simulink model "NonSimplifiedMBFRC"  (R2023b)
settings: Solver=FixedStepAuto  StartTime=0.0  StopTime=t(end)  FixedStep=0.001  MaxStep=0.001  RelTol=1e-3
values from neighbouring files (symbols this model uses):
  a = 0.02+(j-1)*0.02    [MBFRC_ForLoops.m]    (also in Main.m = 0.001)
  f = f3    [MBFRC_ForLoops.m]    (also in Main.m = [0 freqs(1:Nfreqs)])
  phi_mat = zeros(2*length(f))    [MBFRC_ForLoops.m]    (also in Main.m)
  pQ = nQ    (= 12)    [MBFRC_ForLoops.m]    (also in Main.m)
  refOn = 1    [MBFRC_ForLoops.m]    (also in Main.m)
  tradRC_on = 1    [Main.m]
undefined symbols (not defined in the file or in its folder): phd, r_scale, tau
libraries: cstblocks x5
settings Model: Creator=maxja  LastModifiedBy=maxja

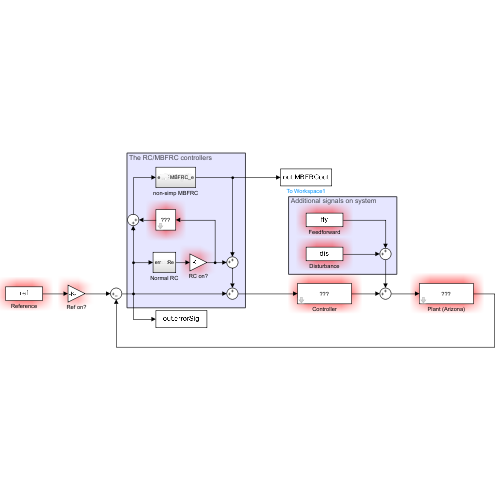
[thumbnail: Simulink's stored preview of the top-level diagram]
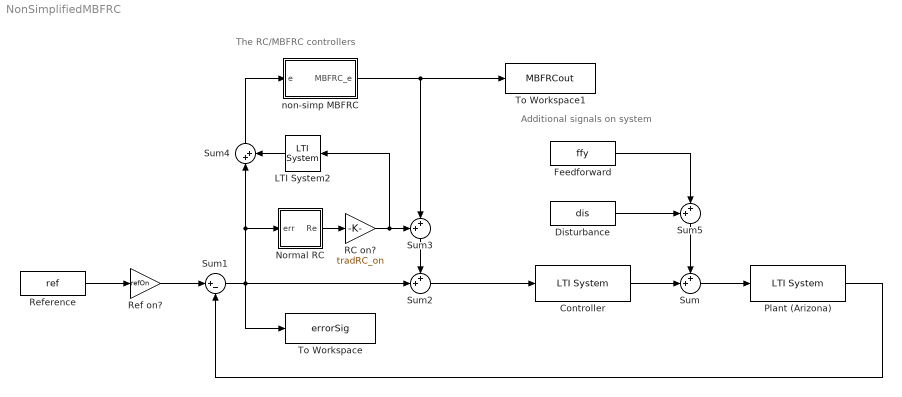
== system NonSimplifiedMBFRC ==
  note: Additional signals on system
  note: The RC/MBFRC controllers
  Controller : cstblocks/LTI System  sys=Cz  IC=[]  PadeOrder=0
  Disturbance : FromWorkspace  VariableName=dis
  Feedforward : FromWorkspace  VariableName=ffy
  LTI System2 : cstblocks/LTI System  sys=T  IC=[]  PadeOrder=0
  Normal RC : Subsystem
  Plant (Arizona) : cstblocks/LTI System  sys=Pz  IC=[]  PadeOrder=0
  RC on? : Gain  Gain=tradRC_on
  Ref on? : Gain  Gain=refOn
  Reference : FromWorkspace  VariableName=ref
  Sum{,2..3,5} (4 alike) : Sum  Inputs=++|
  Sum1 : Sum  Inputs=|+-
  Sum4 : Sum  Inputs=|++
  To Workspace : ToWorkspace  VariableName=errorSig  SaveFormat=Timeseries  SampleTime=-1
  To Workspace1 : ToWorkspace  VariableName=MBFRCout  SaveFormat=Timeseries  SampleTime=-1
  non-simp MBFRC : Subsystem
  wires:
  Controller/1 -> Sum/2
  Reference/1 -> Ref on?/1
  Plant (Arizona)/1 -> Sum1/2
  Sum2/1 -> Controller/1
  non-simp MBFRC/1(MBFRC_e) -> Sum3/2, To Workspace1/1
  LTI System2/1 -> Sum4/2
  Sum4/1 -> non-simp MBFRC/1(e)
  Normal RC/1(Re) -> RC on?/1
  Sum1/1 -> To Workspace/1, Sum2/2, Sum4/1, Normal RC/1(err)
  Sum3/1 -> Sum2/1
  Sum/1 -> Plant (Arizona)/1
  Disturbance/1 -> Sum5/1
  Ref on?/1 -> Sum1/1
  Feedforward/1 -> Sum5/2
  Sum5/1 -> Sum/1
  RC on?/1 -> Sum3/1, LTI System2/1

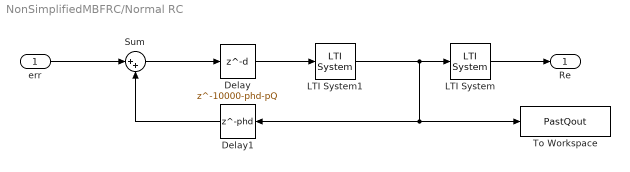
== system NonSimplifiedMBFRC/Normal RC ==
  err : Inport
  Delay : Delay  DelayLength=10000-phd-pQ
  Delay1 : Delay  DelayLength=phd
  LTI System : cstblocks/LTI System  sys=Lc  IC=[]  PadeOrder=0
  LTI System1 : cstblocks/LTI System  sys=Qc  IC=[]  PadeOrder=0
  Sum : Sum  Inputs=|++
  To Workspace : ToWorkspace  VariableName=PastQout  SaveFormat=Timeseries  SampleTime=-1
  Re : Outport
  wires:
  err/1 -> Sum/1
  Sum/1 -> Delay/1
  Delay/1 -> LTI System1/1
  LTI System/1 -> Re/1
  Delay1/1 -> Sum/2
  LTI System1/1 -> To Workspace/1, Delay1/1, LTI System/1

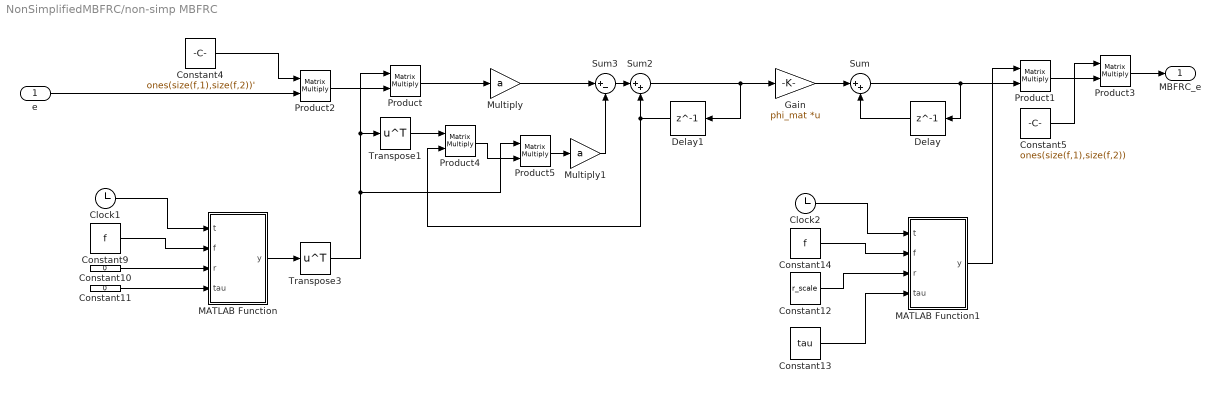
== system NonSimplifiedMBFRC/non-simp MBFRC ==
  e : Inport
  Clock1 : Clock
  Clock2 : Clock
  Constant10 : Constant  Value=0
  Constant11 : Constant  Value=0
  Constant12 : Constant  Value=r_scale
  Constant13 : Constant  Value=tau
  Constant14 : Constant  Value=f
  Constant4 : Constant  Value=ones(size(f,1),size(f,2))'  VectorParams1D=off
  Constant5 : Constant  Value=ones(size(f,1),size(f,2))  VectorParams1D=off
  Constant9 : Constant  Value=f
  Delay : Delay  DelayLength=1
  Delay1 : Delay  DelayLength=1
  Gain : Gain  Gain=phi_mat  Multiplication=Matrix(K*u)
  MATLAB Function : MATLAB Function  TreatAsAtomicUnit=on
  MATLAB Function1 : MATLAB Function  TreatAsAtomicUnit=on
  Multiply : Gain  Gain=a
  Multiply1 : Gain  Gain=a
  Product{,1..5} (6 alike) : Product  Multiplication=Matrix(*)
  Sum : Sum  Inputs=|++
  Sum2 : Sum  Inputs=|++
  Sum3 : Sum  Inputs=|+-
  Transpose1 : Math  Operator=transpose
  Transpose3 : Math  Operator=transpose
  MBFRC_e : Outport
  wires:
  Sum2/1 -> Gain/1, Delay1/1
  Gain/1 -> Sum/1
  Delay/1 -> Sum/2
  Sum/1 -> Delay/1, Product1/2
  Constant4/1 -> Product2/1
  e/1 -> Product2/2
  Product2/1 -> Product/2
  Product3/1 -> MBFRC_e/1
  Product1/1 -> Product3/2
  Clock1/1 -> MATLAB Function/1(t)
  MATLAB Function/1(y) -> Transpose3/1
  Constant9/1 -> MATLAB Function/2(f)
  Constant10/1 -> MATLAB Function/3(r)
  Constant11/1 -> MATLAB Function/4(tau)
  Constant14/1 -> MATLAB Function1/2(f)
  Constant13/1 -> MATLAB Function1/4(tau)
  Constant12/1 -> MATLAB Function1/3(r)
  Clock2/1 -> MATLAB Function1/1(t)
  MATLAB Function1/1(y) -> Product1/1
  Sum3/1 -> Sum2/1
  Delay1/1 -> Sum2/2, Product4/2
  Multiply/1 -> Sum3/1
  Product/1 -> Multiply/1
  Transpose1/1 -> Product4/1
  Product5/1 -> Multiply1/1
  Multiply1/1 -> Sum3/2
  Product4/1 -> Product5/2
  Transpose3/1 -> Product5/1, Product/1, Transpose1/1
  Constant5/1 -> Product3/1

== matlab function NonSimplifiedMBFRC/non-simp MBFRC/MATLAB Function1 ==
  data: t input; y output; f input; r input; tau input
function y = fcn(t,f,r,tau)

[n,~] = size(f);

y = zeros(n,2*n);

for i=1:n
    if f(i) ~=0
        y(i,2*(i-1)+1) = 1/r(i)*cos(f(i)*2*pi*t-tau(i)*pi/180);
        y(i,2*(i-1)+2) = 1/r(i)*sin(f(i)*2*pi*t-tau(i)*pi/180);
    else
        y(i,2*(i-1)+1) = 1/r(i)*1;
        y(i,2*(i-1)+2) = 0;
    end
end

== matlab function NonSimplifiedMBFRC/non-simp MBFRC/MATLAB Function ==
  data: t input; y output; f input; r input; tau input
function y = fcn(t,f,r,tau)

[n,~] = size(f);

y = zeros(n,2*n);

for i=1:n
    if f(i) ~= 0
        y(i,2*(i-1)+1) = cos(f(i)*2*pi*t);
        y(i,2*(i-1)+2) = sin(f(i)*2*pi*t);
    else
        y(i,2*(i-1)+1) = 1;
        y(i,2*(i-1)+2) = 0;
    end
end
